simulink model "item1PS"  (R2017a)
settings: Solver=VariableStepAuto  StartTime=0.0  StopTime=30  RelTol=1e-3
settings Model: Creator=julia  LastModifiedBy=julia

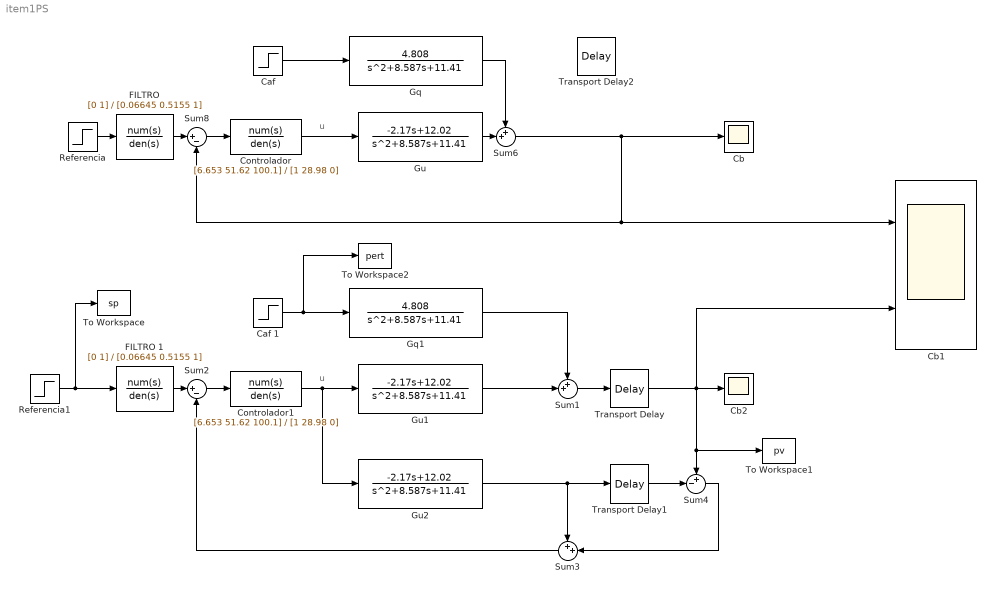
== system item1PS ==
  note: u
  note: u
  "    Controlador" : TransferFcn  Numerator=[6.653 51.62 100.1]  Denominator=[1 28.98 0]
  "    Controlador1" : TransferFcn  Numerator=[6.653 51.62 100.1]  Denominator=[1 28.98 0]
  "Caf " : Step  Time=20  After=0.5  SampleTime=0
  Caf 1 : Step  Time=20  After=0.5  SampleTime=0
  Cb : Scope
  Cb1 : Scope  NumInputPorts=2
  Cb2 : Scope
  "FILTRO " : TransferFcn  Numerator=[0 1]  Denominator=[0.06645 0.5155 1]
  FILTRO 1 : TransferFcn  Numerator=[0 1]  Denominator=[0.06645 0.5155 1]
  Gq : TransferFcn  Numerator=[0 4.808]  Denominator=[1 8.587 11.41]
  Gq1 : TransferFcn  Numerator=[0 4.808]  Denominator=[1 8.587 11.41]
  Gu : TransferFcn  Numerator=[-2.17 12.02]  Denominator=[1 8.587 11.41]
  Gu1 : TransferFcn  Numerator=[-2.17 12.02]  Denominator=[1 8.587 11.41]
  Gu2 : TransferFcn  Numerator=[-2.17 12.02]  Denominator=[1 8.587 11.41]
  Referencia : Step  Time=0  SampleTime=0
  Referencia1 : Step  Time=0  SampleTime=0
  Sum1 : Sum  Inputs=++|
  Sum2 : Sum  Inputs=|+-
  Sum3 : Sum  Inputs=++|
  Sum4 : Sum  Inputs=+-|
  Sum6 : Sum  Inputs=++|
  Sum8 : Sum  Inputs=|+-
  To Workspace : ToWorkspace  VariableName=sp  SaveFormat=Timeseries  SampleTime=-1
  To Workspace1 : ToWorkspace  VariableName=pv  SaveFormat=Timeseries  SampleTime=-1
  To Workspace2 : ToWorkspace  VariableName=pert  SaveFormat=Timeseries  SampleTime=-1
  Transport Delay : TransportDelay  DelayTime=3
  Transport Delay1 : TransportDelay  DelayTime=3
  Transport Delay2 : TransportDelay  DelayTime=3
  wires:
  "Caf "/1 -> Gq/1
  Gq/1 -> Sum6/1
  Sum8/1 -> "    Controlador"/1
  Gu/1 -> Sum6/2
  "    Controlador"/1 -> Gu/1
  Referencia/1 -> "FILTRO "/1
  "FILTRO "/1 -> Sum8/1
  FILTRO 1/1 -> Sum2/1
  Referencia1/1 -> To Workspace/1, FILTRO 1/1
  "    Controlador1"/1 -> Gu2/1, Gu1/1
  Gu1/1 -> Sum1/2
  Sum2/1 -> "    Controlador1"/1
  Gq1/1 -> Sum1/1
  Caf 1/1 -> To Workspace2/1, Gq1/1
  Sum1/1 -> Transport Delay/1
  Gu2/1 -> Sum3/1, Transport Delay1/1
  Sum3/1 -> Sum2/2
  Transport Delay1/1 -> Sum4/2
  Sum4/1 -> Sum3/2
  Transport Delay/1 -> Cb1/2, Cb2/1, To Workspace1/1, Sum4/1
  Sum6/1 -> Cb1/1, Sum8/2, Cb/1
